simulink model "PD_sim_3_5"  (R2018b)
settings: Solver=FixedStepAuto  StartTime=0.0  StopTime=10.0  FixedStep=0.001  RelTol=1e-3
settings Model: Creator=robolux  LastModifiedBy=robolux

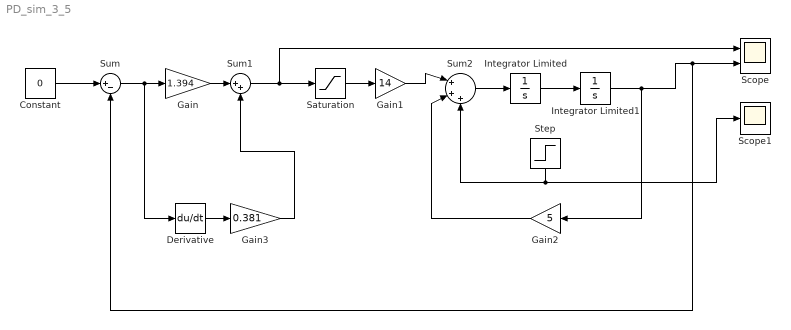
== system PD_sim_3_5 ==
  Constant : Constant  Value=0
  Derivative : Derivative
  Gain : Gain  Gain=1.394
  Gain1 : Gain  Gain=14
  Gain2 : Gain  Gain=5
  Gain3 : Gain  Gain=0.381
  Integrator Limited : Integrator  InitialCondition=0.5  LimitOutput=on  UpperSaturationLimit=pi/6  LowerSaturationLimit=-pi/6
  Integrator Limited1 : Integrator  InitialCondition=0.1  LimitOutput=on  UpperSaturationLimit=pi/6  LowerSaturationLimit=-pi/6
  Saturation : Saturate  UpperLimit=pi/6  LowerLimit=-pi/6
  Scope : Scope  NumInputPorts=2
  Scope1 : Scope
  Step : Step  Time=4  After=3.5  SampleTime=0
  Sum : Sum  Inputs=|+-
  Sum1 : Sum  Inputs=|++
  Sum2 : Sum  Inputs=|+++
  wires:
  Sum/1 -> Derivative/1, Gain/1
  Integrator Limited/1 -> Integrator Limited1/1
  Derivative/1 -> Gain3/1
  Sum2/1 -> Integrator Limited/1
  Integrator Limited1/1 -> Gain2/1, Scope/2, Sum/2
  Gain2/1 -> Sum2/2
  Gain1/1 -> Sum2/1
  Constant/1 -> Sum/1
  Saturation/1 -> Gain1/1
  Gain3/1 -> Sum1/2
  Sum1/1 -> Scope/1, Saturation/1
  Gain/1 -> Sum1/1
  Step/1 -> Sum2/3, Scope1/1
